simulink library "LopesDevelopmentLibrary"  (R2015b)
settings: Solver=ode45  StartTime=0.0  StopTime=10.0  RelTol=1e-3
values from neighbouring files (symbols this model uses):
  d2r = @(d) d*(pi/180)    [LopesDevelopmentLibrary_LoadParameters.m]
  ts = LopesParams.ts    [LopesDevelopmentLibrary_LoadParameters.m]
undefined symbols (not defined in the file or in its folder): anyParameterChanged, DiscIntNeverNeededParam, gcbh, LAP, LHF, LKF, LopesParams, macaddr, mxpcnetworkconfig, mxpcrtudprx, mxpcrtudptx, patientParametersChanged, port, PX, PZ, RAP, RHF, RKF, SelectorLOPESInSize, StrideTime_s, Time
undefined symbols (not defined in the file): LopesParamsSendDataArrayLen
libraries: LopesDevelopmentLibrary x327, simulink x100, dspmtrx3 x49, xpciplib x6, xpcnetworkbufferlib x5, dspsigops x4, dspstat3 x3, xpcethernetlib x2, visionstatistics x2, xpcseriallib x2, LopesDevelopmentLibraryTest x1, nmc x1
(part 4 of 12)

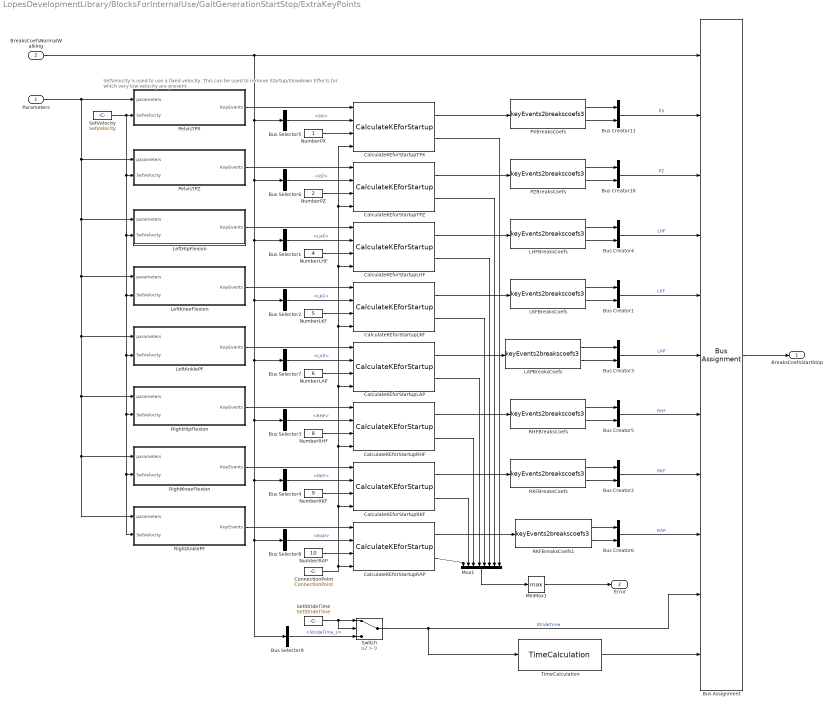
== system LopesDevelopmentLibrary/BlocksForInternalUse/GaitGenerationStartStop/ExtraKeyPoints  ==
  note: SetVelocity is used to use a fixed velocity.
      | This can be used to remove Startup/Slowdown Effects for which very low velocity are present
  Parameters : Inport
  BreaksCoefsNormalWalking : Inport  Port=2
  Bus Creator{1..6,10..11} (8 alike) : BusCreator  Inputs=2
  Bus Selector1 : BusSelector  OutputSignals=LHF
  Bus Selector2 : BusSelector  OutputSignals=LKF
  Bus Selector3 : BusSelector  OutputSignals=RHF
  Bus Selector4 : BusSelector  OutputSignals=RKF
  Bus Selector5 : BusSelector  OutputSignals=PX
  Bus Selector6 : BusSelector  OutputSignals=PZ
  Bus Selector7 : BusSelector  OutputSignals=LAP
  Bus Selector8 : BusSelector  OutputSignals=RAP
  Bus Selector9 : BusSelector  OutputSignals=StrideTime_s
  Bus Assignment : BusAssignment  AssignedSignals=PX,PZ,LHF,LKF,LAP,RHF,RKF,RAP,StrideTime_s,Time
  CalculateKEforStartupLAP : LopesDevelopmentLibrary/BlocksForInternalUse/GaitGenerationStartStop/CalculateKEforStartup
  CalculateKEforStartupLHF : LopesDevelopmentLibrary/BlocksForInternalUse/GaitGenerationStartStop/CalculateKEforStartup
  CalculateKEforStartupLKF : LopesDevelopmentLibrary/BlocksForInternalUse/GaitGenerationStartStop/CalculateKEforStartup
  CalculateKEforStartupRAP : LopesDevelopmentLibrary/BlocksForInternalUse/GaitGenerationStartStop/CalculateKEforStartup
  CalculateKEforStartupRHF : LopesDevelopmentLibrary/BlocksForInternalUse/GaitGenerationStartStop/CalculateKEforStartup
  CalculateKEforStartupRKF : LopesDevelopmentLibrary/BlocksForInternalUse/GaitGenerationStartStop/CalculateKEforStartup
  CalculateKEforStartupTPX : LopesDevelopmentLibrary/BlocksForInternalUse/GaitGenerationStartStop/CalculateKEforStartup
  CalculateKEforStartupTPZ : LopesDevelopmentLibrary/BlocksForInternalUse/GaitGenerationStartStop/CalculateKEforStartup
  ConnectionPoint : Constant  Value=ConnectionPoint
  LAPBreaksCoefs : LopesDevelopmentLibrary/BlocksForInternalUse/GaitGeneration/keyEvents2breakscoefs3  SystemSampleTime=-1
  LHFBreaksCoefs : LopesDevelopmentLibrary/BlocksForInternalUse/GaitGeneration/keyEvents2breakscoefs3  SystemSampleTime=-1
  LKFBreaksCoefs : LopesDevelopmentLibrary/BlocksForInternalUse/GaitGeneration/keyEvents2breakscoefs3  SystemSampleTime=-1
  LeftAnklePF : Subsystem
  LeftHipFlexion : Subsystem
  LeftKneeFlexion : Subsystem
  MinMax1 : MinMax  Function=max
  Mux1 : Mux  Inputs=8
  NumberLAP : Constant  Value=6
  NumberLHF : Constant  Value=4
  NumberLKF : Constant  Value=5
  NumberPX : Constant
  NumberPZ : Constant  Value=2
  NumberRAP : Constant  Value=10
  NumberRHF : Constant  Value=8
  NumberRKF : Constant  Value=9
  PXBreaksCoefs : LopesDevelopmentLibrary/BlocksForInternalUse/GaitGeneration/keyEvents2breakscoefs3  SystemSampleTime=-1
  PZBreaksCoefs : LopesDevelopmentLibrary/BlocksForInternalUse/GaitGeneration/keyEvents2breakscoefs3  SystemSampleTime=-1
  PelvisTPX : Subsystem
  PelvisTPZ : Subsystem
  RHFBreaksCoefs : LopesDevelopmentLibrary/BlocksForInternalUse/GaitGeneration/keyEvents2breakscoefs3  SystemSampleTime=-1
  RKFBreaksCoefs : LopesDevelopmentLibrary/BlocksForInternalUse/GaitGeneration/keyEvents2breakscoefs3  SystemSampleTime=-1
  RKFBreaksCoefs1 : LopesDevelopmentLibrary/BlocksForInternalUse/GaitGeneration/keyEvents2breakscoefs3  SystemSampleTime=-1
  RightAnklePF : Subsystem
  RightHipFlexion : Subsystem
  RightKneeFlexion : Subsystem
  SetStrideTime : Constant  Value=SetStrideTime
  SetVelocity : Constant  Value=SetVelocity
  Switch : Switch  Criteria=u2 > Threshold
  TimeCalculation : LopesDevelopmentLibraryTest/BlocksForInternalUse/GaitGenerationStartStop/ExtraKeyPoints /TimeCalculation
  BreaksCoefsStartStop : Outport
  Error : Outport  Port=2
  wires:
  Switch/1 -> TimeCalculation/1, Bus Assignment/10  "StrideTime"
  BreaksCoefsNormalWalking/1 -> Bus Assignment/1, Bus Selector5/1, Bus Selector6/1, Bus Selector7/1, Bus Selector4/1, Bus Selector8/1, Bus Selector9/1, Bus Selector3/1, Bus Selector2/1, Bus Selector1/1
  Bus Selector9/1 -> Switch/3  "<StrideTime_s>"
  SetStrideTime/1 -> Switch/2, Switch/1
  TimeCalculation/1 -> Bus Assignment/11
  Parameters/1 -> PelvisTPX/1(parameters), PelvisTPZ/1(parameters), LeftHipFlexion/1(parameters), LeftKneeFlexion/1(parameters), LeftAnklePF/1(parameters), RightHipFlexion/1(parameters), RightKneeFlexion/1(parameters), RightAnklePF/1(parameters)
  RightAnklePF/1(KeyEvents) -> CalculateKEforStartupRAP/1
  NumberRAP/1 -> CalculateKEforStartupRAP/3
  Bus Selector8/1 -> CalculateKEforStartupRAP/2  "<RAP>"
  CalculateKEforStartupRAP/1 -> RKFBreaksCoefs1/1
  Bus Creator6/1 -> Bus Assignment/9  "RAP"
  RKFBreaksCoefs1/2 -> Bus Creator6/2
  RKFBreaksCoefs1/1 -> Bus Creator6/1
  Bus Creator3/1 -> Bus Assignment/6  "LAP"
  LAPBreaksCoefs/2 -> Bus Creator3/2
  LAPBreaksCoefs/1 -> Bus Creator3/1
  CalculateKEforStartupLAP/1 -> LAPBreaksCoefs/1
  Bus Selector7/1 -> CalculateKEforStartupLAP/2  "<LAP>"
  LeftAnklePF/1(KeyEvents) -> CalculateKEforStartupLAP/1
  NumberLAP/1 -> CalculateKEforStartupLAP/3
  Bus Assignment/1 -> BreaksCoefsStartStop/1
  ConnectionPoint/1 -> CalculateKEforStartupRKF/4, CalculateKEforStartupLKF/4, CalculateKEforStartupTPX/4, CalculateKEforStartupTPZ/4, CalculateKEforStartupLHF/4, CalculateKEforStartupLAP/4, CalculateKEforStartupRHF/4, CalculateKEforStartupRAP/4
  Bus Creator2/1 -> Bus Assignment/8  "RKF"
  Bus Creator5/1 -> Bus Assignment/7  "RHF"
  Bus Creator1/1 -> Bus Assignment/5  "LKF"
  CalculateKEforStartupLHF/2 -> Mux1/6
  CalculateKEforStartupLKF/2 -> Mux1/5
  CalculateKEforStartupRHF/2 -> Mux1/3
  CalculateKEforStartupRKF/2 -> Mux1/2
  CalculateKEforStartupLHF/1 -> LHFBreaksCoefs/1
  RightKneeFlexion/1(KeyEvents) -> CalculateKEforStartupRKF/1
  LeftKneeFlexion/1(KeyEvents) -> CalculateKEforStartupLKF/1
  RightHipFlexion/1(KeyEvents) -> CalculateKEforStartupRHF/1
  NumberRKF/1 -> CalculateKEforStartupRKF/3
  NumberRHF/1 -> CalculateKEforStartupRHF/3
  NumberLKF/1 -> CalculateKEforStartupLKF/3
  Bus Selector1/1 -> CalculateKEforStartupLHF/2  "<LHF>"
  LeftHipFlexion/1(KeyEvents) -> CalculateKEforStartupLHF/1
  NumberLHF/1 -> CalculateKEforStartupLHF/3
  CalculateKEforStartupRKF/1 -> RKFBreaksCoefs/1
  CalculateKEforStartupLKF/1 -> LKFBreaksCoefs/1
  CalculateKEforStartupRHF/1 -> RHFBreaksCoefs/1
  Bus Creator4/1 -> Bus Assignment/4  "LHF"
  Bus Selector4/1 -> CalculateKEforStartupRKF/2  "<RKF>"
  Bus Selector3/1 -> CalculateKEforStartupRHF/2  "<RHF>"
  Bus Selector2/1 -> CalculateKEforStartupLKF/2  "<LKF>"
  LKFBreaksCoefs/2 -> Bus Creator1/2
  RKFBreaksCoefs/2 -> Bus Creator2/2
  LKFBreaksCoefs/1 -> Bus Creator1/1
  RKFBreaksCoefs/1 -> Bus Creator2/1
  LHFBreaksCoefs/2 -> Bus Creator4/2
  RHFBreaksCoefs/2 -> Bus Creator5/2
  RHFBreaksCoefs/1 -> Bus Creator5/1
  LHFBreaksCoefs/1 -> Bus Creator4/1
  Mux1/1 -> MinMax1/1
  MinMax1/1 -> Error/1
  SetVelocity/1 -> PelvisTPX/2(SetVelocity), PelvisTPZ/2(SetVelocity), LeftAnklePF/2(SetVelocity), RightHipFlexion/2(SetVelocity), RightKneeFlexion/2(SetVelocity), RightAnklePF/2(SetVelocity), LeftKneeFlexion/2(SetVelocity), LeftHipFlexion/2(SetVelocity)
  CalculateKEforStartupTPX/1 -> PXBreaksCoefs/1
  CalculateKEforStartupTPZ/1 -> PZBreaksCoefs/1
  NumberPZ/1 -> CalculateKEforStartupTPZ/3
  PelvisTPX/1(KeyEvents) -> CalculateKEforStartupTPX/1
  PelvisTPZ/1(KeyEvents) -> CalculateKEforStartupTPZ/1
  NumberPX/1 -> CalculateKEforStartupTPX/3
  Bus Selector5/1 -> CalculateKEforStartupTPX/2  "<PX>"
  Bus Selector6/1 -> CalculateKEforStartupTPZ/2  "<PZ>"
  PXBreaksCoefs/1 -> Bus Creator11/1
  PXBreaksCoefs/2 -> Bus Creator11/2
  PZBreaksCoefs/1 -> Bus Creator10/1
  PZBreaksCoefs/2 -> Bus Creator10/2
  Bus Creator10/1 -> Bus Assignment/3  "PZ"
  Bus Creator11/1 -> Bus Assignment/2  "PX"
  CalculateKEforStartupTPZ/2 -> Mux1/7
  CalculateKEforStartupTPX/2 -> Mux1/8
  CalculateKEforStartupRAP/2 -> Mux1/1
  CalculateKEforStartupLAP/2 -> Mux1/4

== system LopesDevelopmentLibrary/BlocksForInternalUse/GaitGenerationStartStop/OrderKeyEventsAddOne ==
  kE : Inport
  JointNumber : Inport  Port=2
  phase : Inport  Port=3
  yy : Inport  Port=4
  dydx : Inport  Port=5
  SortAndAddKeyEvents : MATLAB Function  TreatAsAtomicUnit=on
  kE_out : Outport
  isError : Outport  Port=2
  wires:
  dydx/1 -> SortAndAddKeyEvents/5(dydx)
  yy/1 -> SortAndAddKeyEvents/4(yy)
  phase/1 -> SortAndAddKeyEvents/3(phase)
  SortAndAddKeyEvents/1(kE_out) -> kE_out/1
  SortAndAddKeyEvents/2(Error) -> isError/1
  kE/1 -> SortAndAddKeyEvents/1(kE)
  JointNumber/1 -> SortAndAddKeyEvents/2(jointNumber)

== system LopesDevelopmentLibrary/BlocksForInternalUse/LLC Communication/LLC Network Configuration ==
  note: This block initializes the separate network card in
      | the (real) xPC Target. When built for usage with the
      | Virtual Machine version (LopesUseRealTimeUDP=0),
      | this block does nothing.
  Dummy : Terminator
  Dummy1 : Constant
  Variant Network Init : Subsystem  Variant=on
  wires:
  Variant Network Init/1(Dummy_out) -> Dummy/1
  Dummy1/1 -> Variant Network Init/1(Dummy_in)

== system LopesDevelopmentLibrary/BlocksForInternalUse/LLC Communication/LLCReceiveUDP ==
  Enable : EnablePort
  Constant3 : Constant  Value=uint8(['Recv ',num2str(port),': '])
  Debug : Subsystem
      mask Display: disp('')
  Dummy1 : Constant  Value=0
  EnableDebug : Constant  Value=false  OutDataTypeStr=boolean
      settings: OpenFcn=|
      | b = get_param(gcb,'value');
      | if (strcmp(b,'true')),
      |   set_param (gcb,'value','false');
      | else
      |   set_param(gcb,'value','true');
      | end;
  ShowInMatlabConsoleIfNotEmpty : MATLAB Function  TreatAsAtomicUnit=on
  UDPReceiveVariantChannel : Subsystem  Variant=on
  RecvData : Outport
  RecvLen : Outport  Port=2
  wires:
  Dummy1/1 -> UDPReceiveVariantChannel/1(Dummy_in)
  Constant3/1 -> ShowInMatlabConsoleIfNotEmpty/3(pre)
  UDPReceiveVariantChannel/1(RecvData) -> RecvData/1, ShowInMatlabConsoleIfNotEmpty/1(stringArray)
  EnableDebug/1 -> ShowInMatlabConsoleIfNotEmpty/4(enable)
  UDPReceiveVariantChannel/2(RecvLen) -> RecvLen/1, ShowInMatlabConsoleIfNotEmpty/2(len)

== system LopesDevelopmentLibrary/BlocksForInternalUse/LLC Communication/LLCSendUDP ==
  SendData : Inport
  SendLen : Inport  Port=2
  Enable : EnablePort
  Compare To Zero : simulink/Logic and Bit Operations/Compare To Zero  relop=>  OutDataTypeStr=boolean
  Constant6 : Constant  Value=uint8(['Send ',num2str(port),': '])
  Debug : Subsystem
      mask Display: disp('')
  EnableDebug : Constant  Value=false  OutDataTypeStr=boolean
      settings: OpenFcn=|
      | b = get_param(gcb,'value');
      | if (strcmp(b,'true')),
      |   set_param (gcb,'value','false');
      | else
      |   set_param(gcb,'value','true');
      | end;
  ShowInMatlabConsole IfNotEmpty : MATLAB Function  TreatAsAtomicUnit=on
  UDPSendVariant : Subsystem
  wires:
  Constant6/1 -> ShowInMatlabConsole IfNotEmpty/3(pre)
  EnableDebug/1 -> ShowInMatlabConsole IfNotEmpty/4(enable)
  SendData/1 -> UDPSendVariant/1(Data), ShowInMatlabConsole IfNotEmpty/1(stringArray)
  Compare To Zero/1 -> UDPSendVariant/Enable
  SendLen/1 -> Compare To Zero/1, UDPSendVariant/2(Len), ShowInMatlabConsole IfNotEmpty/2(len)

== system LopesDevelopmentLibrary/BlocksForInternalUse/LLC Communication/UDP_Blocks ==
  note: These blocks are copies of the UDP blocks (as of R2015b: Legacy UDP) for non-realtime and the RealTime UDP blocks of the xPC/SLRT libraries of different Matlab versions. copied them and disabled/broke the links to the original libraries (needed for the second bullet below). They differ from the original blocks in the Library on the following points:
      | I changed the mask. Foar these blocks, the IP address _is_ evaluated (for the standard blocks it is not). This allows for usage of a variable as IP address (it should be a string).I reduced the receive buffering settings so that always the most recent packet is received (the older ones are discarded).
  "Network Configuration_RT_2012b " : Subsystem  mask(xpcnwconfig){IpAddress=LopesParams.Communication.ipSelf_RT, SubnetMask=255.255.255.0, Gateway=0.0.0.0, EthDrv=Intel Gigabit, PciBus=LopesParams.Communication.busSelf_RT, PciSlot=LopesParams.Communication.slotSelf_RT}
      mask prompts: IpAddress "IP Address:"; SubnetMask "Subnet Mask:"; EthDrv "Ethernet Driver"; PciBus "PCI Bus:"; PciSlot "PCI Slot:"
      mask help: Network Configuration
      mask init:
      | IpAddress = ipaddr(IpAddress);
      | SubnetMask = ipaddr(SubnetMask);
      | Gateway = ipaddr(Gateway);
      mask Help: eval('xpcdoc(''RT_NETWORK_CONFIGURATION'')');
      mask TypeOptions EthDrv: Intel 8255x | Intel Gigabit
      mask Display: disp('Network Configuration');
  "Network Configuration_RT_2014b " : Subsystem  InitFcn=mxpcnetworkconfig(1);  mask(xpcnwconfig){ID=1, IpAddress=LopesParams.Communication.ipSelf_RT, SubnetMask=255.255.255.0, Gateway=0.0.0.0, EthDrv=Intel Gigabit, PciBus=LopesParams.Communication.busSelf_RT, PciSlot=LopesParams.Communication.slotSelf_RT, udpID=0}
      mask prompts: ID "Device ID:"; IpAddress "IP Address:"; SubnetMask "Subnet Mask:"; EthDrv "Ethernet Driver:"; PciBus "PCI Bus:"; PciSlot "PCI Slot:"; udpID "Internal UDP ID:"
      mask help: Configure network interface for real-time UDP communication
      mask init:
      | IpAddress = ipaddr(IpAddress);
      | SubnetMask = ipaddr(SubnetMask);
      | Gateway = ipaddr(Gateway);
      | udpID = ID - 1;
      | 
      | [MaskDisplay] = mxpcnetworkconfig(2, ID, EthDrv, PciBus, PciSlot);
      | set_param(gcb, 'MaskDisplay', MaskDisplay);
      mask Help: eval('xpcdoc(''RT_NETWORK_CONFIGURATION'')');
      mask TypeOptions ID: Ethernet Init /ID
      mask TypeOptions EthDrv: Ethernet Init /Driver
      mask Display: disp('Real-time UDP\nConfiguration\nBus: 2 Slot: 4\nId: 1\nIntel Gigabit');
  Network Configuration_RT_2015b : Subsystem  InitFcn=mxpcnetworkconfig(1);  mask(xpcnwconfig){ID=1, IpAddress=LopesParams.Communication.ipSelf_RT, SubnetMask=255.255.255.0, Gateway=0.0.0.0, EthDrv=Intel Gigabit, PciBus=LopesParams.Communication.busSelf_RT, PciSlot=LopesParams.Communication.slotSelf_RT, udpID=0, MulticastList=[], Multicast={}}
      mask prompts: ID "Device ID:"; IpAddress "IP Address:"; SubnetMask "Subnet Mask:"; EthDrv "Ethernet Driver:"; PciBus "PCI Bus:"; PciSlot "PCI Slot:"; udpID "Internal UDP ID:"; MulticastList "[Multicast IP]"; Multicast "Multicast address list:"
      mask help: Configure network interface for real-time UDP communication.
      mask init: same as LopesDevelopmentLibrary/BlocksForInternalUse/LLC Communication/UDP_Blocks/Network Configuration_RT_2014b 
      mask Help: eval('xpcdoc(''RT_NETWORK_CONFIGURATION'')');
      mask TypeOptions ID: Ethernet Init /ID
      mask TypeOptions EthDrv: Ethernet Init /Driver
      mask TypeOptions MulticastList: ARP Init /MulticastList
      mask TypeOptions Multicast: Ethernet Init /Multicast
      mask Display: disp('Real-time UDP\nConfiguration\nBus: 2 Slot: 4\nId: 1\nIntel Gigabit');
  Receive_Non-RT : S-Function  FunctionName=xpcudpbytereceive  Parameters=ipAdd, ipPort, width, sampletime, vblLen  SFunctionDeploymentMode=off  EnableBusSupport=off  mask(xpcudpbytereceive){ipAddress='0.0.0.0', ipPort=port, width=1500, vblLen=on, sampletime=LopesParams.ts}
      mask prompts: ipAddress "IP address to receive from ('0.0.0.0' for accepting all):"; ipPort "IP port to receive from:"; width "Output port width (number of bytes):"; vblLen "Allow variable length packets"; sampletime "Sample time:"
      mask init:
      | %mudp('ipPort', 'IP Port');
      | ipAdd = ipAddressFromString(ipAddress);
      mask Help: eval('xpcdoc(''UDP_Receive'')');
      mask Display: disp('Non-RT\nUDP Recv\nBinary')
  "Receive_RT_2012b " : Subsystem  mask(receive){Receive1='0.0.0.0', Receive2=port, Receive3=1500, Receive4=LopesParams.ts}
      mask prompts: Receive1 "IP address to receive from ('0.0.0.0' for accepting all):"; Receive2 "IP port to receive from:"; Receive3 "Output port width:"; Receive4 "Sample time:"
      mask init:
      | Receive1 = ipaddr(Receive1);
      mask Help: helpview(fullfile(docroot, 'mapfiles', 'xpc.map'), 'RT_UDP_RECEIVE')
      mask Display: disp('RT UDP\nReceive')
  "Receive_RT_2014b " : Subsystem  InitFcn=mxpcrtudprx(1, get_param(gcbh, 'ID'));  mask(rtudpreceive){ID=1, Receive1='0.0.0.0', Receive2=port, Receive3=1500, Receive4=LopesParams.ts, udpID=0}
      mask prompts: ID "Device ID:"; Receive1 "Source IP Address:"; Receive2 "Local (destination) port:"; Receive3 "Output port width:"; Receive4 "Sample time:"; udpID "Internal UDP ID:"
      mask help:
      | Receive data over UDP network.
      |
      | This block receives data on the specified local (destination) port. To receive all data sent to this port, set 'Source IP Address' to 0.0.0.0. To receive data sent to this port from a specific remote source, enter that IP address.
      mask init:
      | Receive1 = ipaddr(Receive1);
      | udpID = ID -1;
      | [MaskDisplay] = mxpcrtudprx(2, ID);
      | set_param(gcb, 'MaskDisplay', MaskDisplay);
      mask Help: eval('xpcdoc(''RT_UDP_RECEIVE'')');
      mask TypeOptions ID: 1 | 2 | 3 | 4 | 5 | 6 | 7 | 8
      mask Display:
      | disp('UDP\nReceive\nId: 1');
      | port_label('output', 1, 'Data');
      | port_label('output', 2, 'N');
  Receive_RT_2015b : Subsystem  InitFcn=mxpcrtudprx(1, get_param(gcbh, 'ID'));  mask(rtudpreceive){ID=1, Receive1='0.0.0.0', Receive2=port, Receive3=1500, Receive4=LopesParams.ts, udpID=0}
      mask prompts: ID "Device ID:"; Receive1 "Source IP Address:"; Receive2 "Local (destination) port:"; Receive3 "Output port width:"; Receive4 "Sample time:"; udpID "Internal UDP ID:"
      mask help:
      | Receive data over UDP network on a dedicated network interface.
      |
      | This block receives data on the specified local (destination) port. To receive all data sent to this port, set 'Source IP Address' to 0.0.0.0. To receive data sent to this port from a specific remote source, enter the IP address of that source.
      mask init:
      | Receive1 = ipaddr(Receive1);
      | udpID = ID -1;
      | [MaskDisplay] = mxpcrtudprx(2, ID);
      | set_param(gcb, 'MaskDisplay', MaskDisplay);
      mask Help: eval('xpcdoc(''RT_UDP_RECEIVE'')');
      mask TypeOptions ID: 1 | 2 | 3 | 4 | 5 | 6 | 7 | 8
      mask Display:
      | disp('UDP\nReceive\nId: 1');
      | port_label('output', 1, 'Data');
      | port_label('output', 2, 'N');
  Send_Non-RT : S-Function  FunctionName=xpcudpbytesend  Parameters=ipAdd, ipPort, localPort, sampletime, vblLen  SFunctionDeploymentMode=off  EnableBusSupport=off  mask(xpcudpbytesend){ipAddress=LopesParams.Communication.ipLLC_NonRT, ipPort=port, localPort=-1, vblLen=on, sampletime=LopesParams.ts}
      mask prompts: ipAddress "IP address to send to ('255.255.255.255' for broadcast):"; ipPort "Remote IP port to send to:"; localPort "Use the following local IP port (-1 for automatic port assignment):"; vblLen "Allow variable length packets"; sampletime "Sample time:"
      mask init:
      | if localPort ~= -1
      |   mudp('localPort', 'Local IP Port');
      | end
      | ipAdd = ipAddressFromString(ipAddress);
      mask Help: eval('xpcdoc(''UDP_Send'')');
      mask Display: disp('Non-RT\nUDP Send\nBinary')
  Send_RT_2012b : Subsystem  mask(send){Send1=LopesParams.Communication.ipLLC_RT, Send2=port, Send3=-1, Send4=LopesParams.ts}
      mask prompts: Send1 "IP address to send to ('255.255.255.255' for broadcast):"; Send2 "Remote IP port to send to:"; Send3 "Use the following local IP port (-1 for automatic assignment):"; Send4 "Sample time:"
      mask init:
      | Send1 = ipaddr(Send1);
      mask Help: helpview(fullfile(docroot, 'mapfiles', 'xpc.map'), 'RT_UDP_SEND')
      mask Display: disp('RT UDP\nSend')
  Send_RT_2014b : Subsystem  InitFcn=mxpcrtudptx(1, get_param(gcbh, 'ID'));  mask(rtudpsend){ID=1, Send1=LopesParams.Communication.ipLLC_RT, Send2=port, Send3=-1, Send4=LopesParams.ts, udpID=0}
      mask prompts: ID "Device ID:"; Send1 "Destination IP address:"; Send2 "Destination port:"; Send3 "Local (source) port:"; Send4 "Sample time:"; udpID "Internal UDP ID:"
      mask help:
      | Send data over UDP network.
      |
      | This block sends data from the 'Local (source) port' to the 'Destination port'. To broadcast data to 'Destination port' on all devices set 'Destination IP Address' to 255.255.255.255. To send data to a specific remote destintion set that IP address. Set 'Local (source) port' to -1 for automatic assignment.
      mask init:
      | Send1 = ipaddr(Send1);
      | udpID = ID -1;
      | MaskDisplay = mxpcrtudptx(2, ID);
      | set_param(gcb, 'MaskDisplay', MaskDisplay);
      mask Help: eval('xpcdoc(''RT_UDP_SEND'')');
      mask TypeOptions ID: 1 | 2 | 3 | 4 | 5 | 6 | 7 | 8
      mask Display:
      | disp('UDP\nSend\nId: 1');
      | port_label('input', 1, 'Data');
      | port_label('input', 2, 'N');
  Send_RT_2015b : Subsystem  InitFcn=mxpcrtudptx(1, get_param(gcbh, 'ID'));  mask(rtudpsend){ID=1, Send1=LopesParams.Communication.ipLLC_RT, Send2=port, Send3=-1, Send4=LopesParams.ts, udpID=0}
      mask prompts: ID "Device ID:"; Send1 "Destination IP address:"; Send2 "Destination port:"; Send3 "Local (source) port:"; Send4 "Sample time:"; udpID "Internal UDP ID:"
      mask help:
      | Send data over UDP network on a dedicated network interface.
      |
      | This block sends data from the 'Local (source) port' to the 'Destination port'. To broadcast data to 'Destination port' on all devices set 'Destination IP Address' to 255.255.255.255. To send data to a specific remote destintion set that IP address. Set 'Local (source) port' to -1 for automatic assignment.
      mask init:
      | Send1 = ipaddr(Send1);
      | udpID = ID -1;
      | MaskDisplay = mxpcrtudptx(2, ID);
      | set_param(gcb, 'MaskDisplay', MaskDisplay);
      mask Help: eval('xpcdoc(''RT_UDP_SEND'')');
      mask TypeOptions ID: 1 | 2 | 3 | 4 | 5 | 6 | 7 | 8
      mask Display:
      | disp('UDP\nSend\nId: 1');
      | port_label('input', 1, 'Data');
      | port_label('input', 2, 'N');

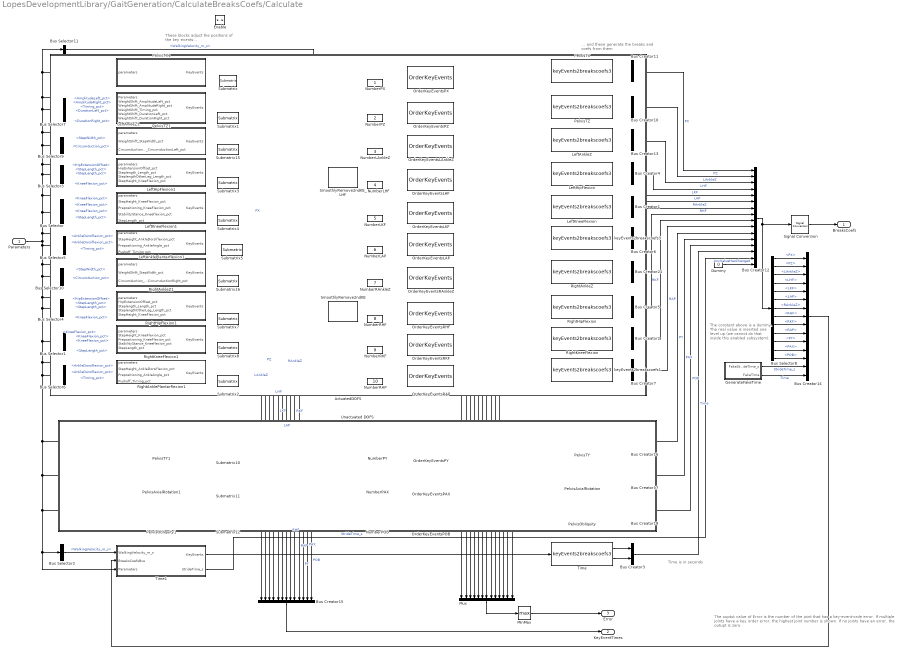
== system LopesDevelopmentLibrary/GaitGeneration/CalculateBreaksCoefs/Calculate ==
  note: The ouptut value of Error is the number of the joint that has a key-event-orde  error.
      | If multiple joints have a key order error, the highest joint number is shown. If
      | no joints have an error, the outupt is zero.
  note: The constant above is
      | a dummy. The real value
      | is inserted one level up
      | (we cannot do that inside this
      | enabled subsystem).
  note: These blocks adjust the positions
      | of the key events...
  note: ... and these generate the breaks
      | and coefs from them
  note: Time is in seconds
  Parameters : Inport
  Enable : EnablePort
  ActuatedDOFS : Subsystem
      mask Display: disp('')
  Bus Creator{1..7,10..11,13,16..18,21} (14 alike) : BusCreator  Inputs=2
  Bus Creator12 : BusCreator  Inputs=16
  Bus Creator14 : BusCreator  Inputs=15
  Bus Creator15 : BusCreator  Inputs=13
  Bus Selector : BusSelector  OutputSignals=LeftStepHeight.KneeFlexion_pct,LeftPrepositioning.KneeFlexion_pct,LeftStabilityStance.KneeFlexion_pct,LeftSteplength.StepLength_pct
  Bus Selector1 : BusSelector  OutputSignals=RightStepHeight.KneeFlexion_pct,RightPrepositioning.KneeFlexion_pct,RightStabilityStance.KneeFlexion_pct,RightSteplength.StepLength_pct
  Bus Selector10 : BusSelector  OutputSignals=WeightShift.StepWidth_pct,RightCircumduction.Circumduction_pct
  Bus Selector11 : BusSelector  OutputSignals=General.WalkingVelocity_m_s
  Bus Selector2 : BusSelector  OutputSignals=General.WalkingVelocity_m_s
  Bus Selector3 : BusSelector  OutputSignals=General.HipExtensionOffset,LeftSteplength.StepLength_pct,RightSteplength.StepLength_pct,LeftStepHeight.KneeFlexion_pct
  Bus Selector4 : BusSelector  OutputSignals=General.HipExtensionOffset,RightSteplength.StepLength_pct,LeftSteplength.StepLength_pct,RightStepHeight.KneeFlexion_pct
  Bus Selector5 : BusSelector  OutputSignals=LeftStepHeight.AnkleDorsiflexion_pct,LeftPrepositioning.AnkleDorsiflexion_pct,LeftPushoff.Timing_pct
  Bus Selector6 : BusSelector  OutputSignals=RightStepHeight.AnkleDorsiflexion_pct,RightPrepositioning.AnkleDorsiflexion_pct,RightPushoff.Timing_pct
  Bus Selector7 : BusSelector  OutputSignals=WeightShift.AmplitudeLeft_pct,WeightShift.AmplitudeRight_pct,WeightShift.Timing_pct,WeightShift.DurationLeft_pct,WeightShift.DurationRight_pct
  Bus Selector8 : BusSelector  OutputSignals=PX,PZ,LAnkleZ,LHF,LKF,LAP,RAnkleZ,RHF,RKF,RAP,PY,PAX,POB
  Bus Selector9 : BusSelector  OutputSignals=WeightShift.StepWidth_pct,LeftCircumduction.Circumduction_pct
  Dummy : Constant  Value=0  OutDataTypeStr=double
  GenerateFakeTime : Subsystem
  LeftAnklePlantarflexion1 : Subsystem
  LeftAnkleZ : LopesDevelopmentLibrary/BlocksForInternalUse/GaitGeneration/keyEvents2breakscoefs3  SystemSampleTime=-1
  LeftAnkleZ1 : Subsystem
  LeftHipFlexion : LopesDevelopmentLibrary/BlocksForInternalUse/GaitGeneration/keyEvents2breakscoefs3  SystemSampleTime=-1
  LeftHipFlexion1 : Subsystem
  LeftKneeFlexion : LopesDevelopmentLibrary/BlocksForInternalUse/GaitGeneration/keyEvents2breakscoefs3  SystemSampleTime=-1
  LeftKneeFlexion1 : Subsystem
  MinMax : MinMax  Function=max
  Mux : Mux  Inputs=13
  NumberLAP : Constant  Value=6
  NumberLAnkleZ : Constant  Value=3
  NumberLHF : Constant  Value=4
  NumberLKF : Constant  Value=5
  NumberPAX : Constant  Value=12
  NumberPOB : Constant  Value=13
  NumberPX : Constant
  NumberPY : Constant  Value=11
  NumberPZ : Constant  Value=2
  NumberRAP : Constant  Value=10
  NumberRAnkleZ : Constant  Value=7
  NumberRHF : Constant  Value=8
  NumberRKF : Constant  Value=9
  OrderKeyEventsLAP : LopesDevelopmentLibrary/BlocksForInternalUse/GaitGeneration/OrderKeyEvents
  OrderKeyEventsLAnkleZ : LopesDevelopmentLibrary/BlocksForInternalUse/GaitGeneration/OrderKeyEvents
  OrderKeyEventsLHF : LopesDevelopmentLibrary/BlocksForInternalUse/GaitGeneration/OrderKeyEvents
  OrderKeyEventsLKF : LopesDevelopmentLibrary/BlocksForInternalUse/GaitGeneration/OrderKeyEvents
  OrderKeyEventsPAX : LopesDevelopmentLibrary/BlocksForInternalUse/GaitGeneration/OrderKeyEvents
  OrderKeyEventsPOB : LopesDevelopmentLibrary/BlocksForInternalUse/GaitGeneration/OrderKeyEvents
  OrderKeyEventsPX : LopesDevelopmentLibrary/BlocksForInternalUse/GaitGeneration/OrderKeyEvents
  OrderKeyEventsPY : LopesDevelopmentLibrary/BlocksForInternalUse/GaitGeneration/OrderKeyEvents
  OrderKeyEventsPZ : LopesDevelopmentLibrary/BlocksForInternalUse/GaitGeneration/OrderKeyEvents
  OrderKeyEventsRAP : LopesDevelopmentLibrary/BlocksForInternalUse/GaitGeneration/OrderKeyEvents
  OrderKeyEventsRAnkleZ : LopesDevelopmentLibrary/BlocksForInternalUse/GaitGeneration/OrderKeyEvents
  OrderKeyEventsRHF : LopesDevelopmentLibrary/BlocksForInternalUse/GaitGeneration/OrderKeyEvents
  OrderKeyEventsRKF : LopesDevelopmentLibrary/BlocksForInternalUse/GaitGeneration/OrderKeyEvents
  PelvisAxialRotation : LopesDevelopmentLibrary/BlocksForInternalUse/GaitGeneration/keyEvents2breakscoefs3  SystemSampleTime=-1
  PelvisAxialRotation1 : Subsystem
  PelvisObliquity : LopesDevelopmentLibrary/BlocksForInternalUse/GaitGeneration/keyEvents2breakscoefs3  SystemSampleTime=-1
  PelvisObliquity1 : Subsystem
  PelvisTX : LopesDevelopmentLibrary/BlocksForInternalUse/GaitGeneration/keyEvents2breakscoefs3  SystemSampleTime=-1
  PelvisTX1 : Subsystem
  PelvisTY : LopesDevelopmentLibrary/BlocksForInternalUse/GaitGeneration/keyEvents2breakscoefs3  SystemSampleTime=-1
  PelvisTY1 : Subsystem
  PelvisTZ : LopesDevelopmentLibrary/BlocksForInternalUse/GaitGeneration/keyEvents2breakscoefs3  SystemSampleTime=-1
  PelvisTZ1 : Subsystem
  RightAnklePlantarflexion1 : Subsystem
  RightAnkleZ : LopesDevelopmentLibrary/BlocksForInternalUse/GaitGeneration/keyEvents2breakscoefs3  SystemSampleTime=-1
  RightAnkleZ1 : Subsystem
  RightHipFlexion : LopesDevelopmentLibrary/BlocksForInternalUse/GaitGeneration/keyEvents2breakscoefs3  SystemSampleTime=-1
  RightHipFlexion1 : Subsystem
  RightKneeFlexion : LopesDevelopmentLibrary/BlocksForInternalUse/GaitGeneration/keyEvents2breakscoefs3  SystemSampleTime=-1
  RightKneeFlexion1 : Subsystem
  Signal Conversion : SignalConversion
  SmoothlyRemove2ndKE : LopesDevelopmentLibrary/BlocksForInternalUse/GaitGeneration/SmoothlyRemove2ndKE
  SmoothlyRemove2ndKE_LHF : LopesDevelopmentLibrary/BlocksForInternalUse/GaitGeneration/SmoothlyRemove2ndKE
  Submatrix{,1..5,7..8,10..12,15..16} (13 alike) : dspmtrx3/Submatrix  RowSpan=All rows  RowStartMode=First  RowStartIndex=1  RowEndMode=Last  RowEndIndex=1  ColSpan=One column  ColStartMode=First  ColStartIndex=1  ColEndMode=Last  ColEndIndex=1
  Time : LopesDevelopmentLibrary/BlocksForInternalUse/GaitGeneration/keyEvents2breakscoefs3  SystemSampleTime=-1
  Time1 : Subsystem
  Unactuated DOFS : Subsystem
      mask Display: disp('')
  keyEvents2breakscoefs1 : LopesDevelopmentLibrary/BlocksForInternalUse/GaitGeneration/keyEvents2breakscoefs3  SystemSampleTime=-1
  keyEvents2breakscoefs3 : LopesDevelopmentLibrary/BlocksForInternalUse/GaitGeneration/keyEvents2breakscoefs3  SystemSampleTime=-1
  BreaksCoefs : Outport  InitialOutput=0
  KeyEventTimes : Outport  Port=2
  Error : Outport  Port=3
  wires:
  Signal Conversion/1 -> BreaksCoefs/1
  OrderKeyEventsRKF/1 -> RightKneeFlexion/1
  OrderKeyEventsLHF/1 -> LeftHipFlexion/1
  Bus Selector7/5 -> PelvisTZ1/6(WeightShift_DurationRight_pct)  "<DurationRight_pct>"
  LeftHipFlexion1/1(KeyEvents) -> SmoothlyRemove2ndKE_LHF/1, Submatrix3/1
  LeftKneeFlexion/2 -> Bus Creator1/2
  LeftHipFlexion/1 -> Bus Creator4/1
  NumberRHF/1 -> OrderKeyEventsRHF/2
  LeftKneeFlexion/1 -> Bus Creator1/1
  MinMax/1 -> Error/1
  NumberRAnkleZ/1 -> OrderKeyEventsRAnkleZ/2
  OrderKeyEventsPOB/1 -> PelvisObliquity/1
  NumberLHF/1 -> OrderKeyEventsLHF/2
  OrderKeyEventsPY/1 -> PelvisTY/1
  NumberPZ/1 -> OrderKeyEventsPZ/2
  OrderKeyEventsPAX/1 -> PelvisAxialRotation/1
  LeftHipFlexion/2 -> Bus Creator4/2
  NumberLKF/1 -> OrderKeyEventsLKF/2
  Bus Selector3/4 -> LeftHipFlexion1/5(StepHeight_KneeFlexion_pct)  "<KneeFlexion_pct>"
  NumberRKF/1 -> OrderKeyEventsRKF/2
  Bus Selector3/3 -> LeftHipFlexion1/4(SteplengthOtherLeg_Length_pct)  "<StepLength_pct>"
  Bus Selector3/2 -> LeftHipFlexion1/3(Steplength_Length_pct)  "<StepLength_pct>"
  Dummy/1 -> Bus Creator12/16  "AnyValueHasChanged"
  RightHipFlexion1/1(KeyEvents) -> Submatrix7/1, SmoothlyRemove2ndKE/1
  Parameters/1 -> Bus Selector5/1, RightAnklePlantarflexion1/1(parameters), Bus Selector6/1, Time1/3(Parameters), Bus Selector2/1, PelvisObliquity1/1(parameters), PelvisAxialRotation1/1(parameters), PelvisTY1/1(parameters), Bus Selector1/1, Bus Selector4/1, RightHipFlexion1/1(parameters), RightKneeFlexion1/1(parameters), Bus Selector10/1, RightAnkleZ1/1(parameters), LeftAnklePlantarflexion1/1(parameters), Bus Selector11/1, PelvisTX1/1(parameters), PelvisTZ1/1(Parameters), Bus Selector7/1, LeftAnkleZ1/1(parameters), Bus Selector9/1, LeftHipFlexion1/1(parameters), Bus Selector3/1, LeftKneeFlexion1/1(parameters), Bus Selector/1
  RightKneeFlexion1/1(KeyEvents) -> OrderKeyEventsRKF/1, Submatrix8/1
  PelvisTX/2 -> Bus Creator11/2
  Bus Creator12/1 -> Signal Conversion/1, Bus Selector8/1
  Bus Creator2/1 -> Bus Creator12/9  "RKF"
  PelvisTX/1 -> Bus Creator11/1
  Bus Creator1/1 -> Bus Creator12/5  "LKF"
  RightHipFlexion/2 -> Bus Creator5/2
  GenerateFakeTime/1(FakeStrideTime_s) -> Bus Creator14/14  "StrideTime_s"
  Bus Selector7/3 -> PelvisTZ1/4(WeightShift_Timing_pct)  "<Timing_pct>"
  LeftKneeFlexion1/1(KeyEvents) -> OrderKeyEventsLKF/1, Submatrix4/1
  Bus Selector7/1 -> PelvisTZ1/2(WeightShift_AmplitudeLeft_pct)  "<AmplitudeLeft_pct>"
  Bus Creator5/1 -> Bus Creator12/8  "RHF"
  Bus Selector7/4 -> PelvisTZ1/5(WeightShift_DurationLeft_pct)  "<DurationLeft_pct>"
  Bus Selector/1 -> LeftKneeFlexion1/2(StepHeight_KneeFlexion_pct)  "<KneeFlexion_pct>"
  Bus Selector4/4 -> RightHipFlexion1/5(StepHeight_KneeFlexion_pct)  "<KneeFlexion_pct>"
  PelvisTX1/1(KeyEvents) -> Submatrix/1, OrderKeyEventsPX/1
  Bus Creator15/1 -> KeyEventTimes/1
  Bus Creator10/1 -> Bus Creator12/2  "PZ"
  Bus Creator11/1 -> Bus Creator12/1  "PX"
  Bus Creator4/1 -> Bus Creator12/4  "LHF"
  Bus Selector4/3 -> RightHipFlexion1/4(SteplengthOtherLeg_Length_pct)  "<StepLength_pct>"
  Bus Selector4/2 -> RightHipFlexion1/3(Steplength_Length_pct)  "<StepLength_pct>"
  PelvisTZ1/1(KeyEvents) -> OrderKeyEventsPZ/1, Submatrix1/1
  PelvisTZ/1 -> Bus Creator10/1
  PelvisTZ/2 -> Bus Creator10/2
  Bus Selector1/4 -> RightKneeFlexion1/5(StepLength_pct)  "<StepLength_pct>"
  SmoothlyRemove2ndKE/1 -> OrderKeyEventsRHF/1
  Bus Selector4/1 -> RightHipFlexion1/2(HipExtensionOffset_pct)  "<HipExtensionOffset>"
  Submatrix10/1 -> Bus Creator15/11  "PY"
  Time1/2(StrideTime_s) -> Bus Creator12/15  "StrideTime_s"
  SmoothlyRemove2ndKE_LHF/1 -> OrderKeyEventsLHF/1
  Bus Selector3/1 -> LeftHipFlexion1/2(HipExtensionOffset_pct)  "<HipExtensionOffset>"
  Bus Selector1/3 -> RightKneeFlexion1/4(StabilityStance_Kneeflexion_pct)  "<KneeFlexion_pct>"
  Bus Selector1/1 -> RightKneeFlexion1/2(StepHeight_KneeFlexion_pct)  "<KneeFlexion_pct>"
  Bus Selector9/2 -> LeftAnkleZ1/3(Circumduction_CircumductionLeft_pct)  "<Circumduction_pct>"
  Bus Selector9/1 -> LeftAnkleZ1/2(WeightShift_StepWidth_pct)  "<StepWidth_pct>"
  NumberLAnkleZ/1 -> OrderKeyEventsLAnkleZ/2
  Bus Selector8/1 -> Bus Creator14/1  "<PX>"
  Bus Selector10/1 -> RightAnkleZ1/2(WeightShift_StepWidth_pct)  "<StepWidth_pct>"
  NumberPX/1 -> OrderKeyEventsPX/2
  Bus Selector10/2 -> RightAnkleZ1/3(Circumduction_CircumductionRight_pct)  "<Circumduction_pct>"
  Bus Selector/4 -> LeftKneeFlexion1/5(StepLength_pct)  "<StepLength_pct>"
  OrderKeyEventsRAnkleZ/1 -> RightAnkleZ/1
  Bus Creator21/1 -> Bus Creator12/7  "RAnkleZ"
  Bus Selector1/2 -> RightKneeFlexion1/3(Prepositioning_KneeFlexion_pct)  "<KneeFlexion_pct>"
  Mux/1 -> MinMax/1
  Bus Selector7/2 -> PelvisTZ1/3(WeightShift_AmplitudeRight_pct)  "<AmplitudeRight_pct>"
  Bus Selector/2 -> LeftKneeFlexion1/3(Prepositioning_KneeFlexion_pct)  "<KneeFlexion_pct>"
  Bus Creator13/1 -> Bus Creator12/3  "LAnkleZ"
  Bus Selector8/2 -> Bus Creator14/2  "<PZ>"
  Bus Selector/3 -> LeftKneeFlexion1/4(StabilityStance_Kneeflexion_pct)  "<KneeFlexion_pct>"
  Bus Selector8/8 -> Bus Creator14/8  "<RHF>"
  LeftAnkleZ/2 -> Bus Creator13/2
  LeftAnkleZ1/1(KeyEvents) -> Submatrix15/1, OrderKeyEventsLAnkleZ/1
  LeftAnkleZ/1 -> Bus Creator13/1
  RightAnkleZ/2 -> Bus Creator21/2
  RightAnkleZ/1 -> Bus Creator21/1
  RightAnkleZ1/1(KeyEvents) -> Submatrix16/1, OrderKeyEventsRAnkleZ/1
  Bus Selector8/12 -> Bus Creator14/12  "<PAX>"
  OrderKeyEventsLAnkleZ/1 -> LeftAnkleZ/1
  Submatrix11/1 -> Bus Creator15/12  "PAX"
  Time/1 -> Bus Creator3/1
  PelvisTY/1 -> Bus Creator16/1
  Bus Selector8/4 -> Bus Creator14/4  "<LHF>"
  Bus Selector8/7 -> Bus Creator14/7  "<RAnkleZ>"
  Bus Selector8/11 -> Bus Creator14/11  "<PY>"
  OrderKeyEventsLAnkleZ/2 -> Mux/3
  Bus Selector8/13 -> Bus Creator14/13  "<POB>"
  Submatrix12/1 -> Bus Creator15/13  "POB"
  Bus Selector8/9 -> Bus Creator14/9  "<RKF>"
  Submatrix8/1 -> Bus Creator15/9  "RKF"
  Submatrix7/1 -> Bus Creator15/8  "RHF"
  Bus Selector8/5 -> Bus Creator14/5  "<LKF>"
  PelvisObliquity1/1(KeyEvents) -> Submatrix12/1, OrderKeyEventsPOB/1
  Bus Selector11/1 -> SmoothlyRemove2ndKE/2, SmoothlyRemove2ndKE_LHF/2  "<WalkingVelocity_m_s>"
  PelvisTY1/1(KeyEvents) -> OrderKeyEventsPY/1, Submatrix10/1
  OrderKeyEventsPZ/2 -> Mux/2
  Submatrix16/1 -> Bus Creator15/7  "RAnkleZ"
  GenerateFakeTime/2(FakeTime) -> Bus Creator14/15  "Time"
  OrderKeyEventsRHF/2 -> Mux/8
  NumberPOB/1 -> OrderKeyEventsPOB/2
  OrderKeyEventsLKF/2 -> Mux/5
  NumberPY/1 -> OrderKeyEventsPY/2
  OrderKeyEventsRAnkleZ/2 -> Mux/7
  Bus Creator16/1 -> Bus Creator12/11  "PY"
  Submatrix/1 -> Bus Creator15/1  "PX"
  Submatrix15/1 -> Bus Creator15/3  "LAnkleZ"
  Submatrix3/1 -> Bus Creator15/4  "LHF"
  Submatrix1/1 -> Bus Creator15/2  "PZ"
  OrderKeyEventsLHF/2 -> Mux/4
  Submatrix4/1 -> Bus Creator15/5  "LKF"
  OrderKeyEventsRKF/2 -> Mux/9
  OrderKeyEventsPY/2 -> Mux/11
  OrderKeyEventsPOB/2 -> Mux/13
  OrderKeyEventsPX/2 -> Mux/1
  OrderKeyEventsPAX/2 -> Mux/12
  Bus Selector8/3 -> Bus Creator14/3  "<LAnkleZ>"
  PelvisTY/2 -> Bus Creator16/2
  OrderKeyEventsRHF/1 -> RightHipFlexion/1
  Time/2 -> Bus Creator3/2
  Bus Creator14/1 -> Time1/2(BreaksCoefsBus)
  RightHipFlexion/1 -> Bus Creator5/1
  OrderKeyEventsPX/1 -> PelvisTX/1
  OrderKeyEventsLKF/1 -> LeftKneeFlexion/1
  OrderKeyEventsPZ/1 -> PelvisTZ/1
  RightKneeFlexion/1 -> Bus Creator2/1
  Time1/1(KeyEvents) -> Time/1
  Bus Selector2/1 -> Time1/1(WalkingVelocity_m_s)  "<WalkingVelocity_m_s>"
  RightKneeFlexion/2 -> Bus Creator2/2
  PelvisObliquity/2 -> Bus Creator18/2
  Bus Creator17/1 -> Bus Creator12/12  "PAX"
  PelvisAxialRotation1/1(KeyEvents) -> Submatrix11/1, OrderKeyEventsPAX/1
  PelvisAxialRotation/2 -> Bus Creator17/2
  PelvisAxialRotation/1 -> Bus Creator17/1
  NumberPAX/1 -> OrderKeyEventsPAX/2
  Bus Creator18/1 -> Bus Creator12/13  "POB"
  PelvisObliquity/1 -> Bus Creator18/1
  Bus Creator3/1 -> Bus Creator12/14  "Time"
  OrderKeyEventsLAP/1 -> keyEvents2breakscoefs3/1
  OrderKeyEventsRAP/1 -> keyEvents2breakscoefs1/1
  keyEvents2breakscoefs3/1 -> Bus Creator6/1
  keyEvents2breakscoefs3/2 -> Bus Creator6/2
  Bus Creator6/1 -> Bus Creator12/6  "LAP"
  keyEvents2breakscoefs1/2 -> Bus Creator7/2
  keyEvents2breakscoefs1/1 -> Bus Creator7/1
  Bus Creator7/1 -> Bus Creator12/10  "RAP"
  Bus Selector8/10 -> Bus Creator14/10  "<RAP>"
  Bus Selector8/6 -> Bus Creator14/6  "<LAP>"
  OrderKeyEventsRAP/2 -> Mux/10
  OrderKeyEventsLAP/2 -> Mux/6
  NumberLAP/1 -> OrderKeyEventsLAP/2
  NumberRAP/1 -> OrderKeyEventsRAP/2
  RightAnklePlantarflexion1/1(KeyEvents) -> Submatrix2/1, OrderKeyEventsRAP/1
  Submatrix2/1 -> Bus Creator15/10  "RAP"
  LeftAnklePlantarflexion1/1(KeyEvents) -> OrderKeyEventsLAP/1, Submatrix5/1
  Submatrix5/1 -> Bus Creator15/6  "LAP"
  Bus Selector5/1 -> LeftAnklePlantarflexion1/2(StepHeight_AnkleDorsiflexion_pct)  "<AnkleDorsiflexion_pct>"
  Bus Selector5/2 -> LeftAnklePlantarflexion1/3(Prepositioning_AnkleAngle_pct)  "<AnkleDorsiflexion_pct>"
  Bus Selector5/3 -> LeftAnklePlantarflexion1/4(Pushoff_Timing_pct)  "<Timing_pct>"
  Bus Selector6/3 -> RightAnklePlantarflexion1/4(Pushoff_Timing_pct)  "<Timing_pct>"
  Bus Selector6/2 -> RightAnklePlantarflexion1/3(Prepositioning_AnkleAngle_pct)  "<AnkleDorsiflexion_pct>"
  Bus Selector6/1 -> RightAnklePlantarflexion1/2(StepHeight_AnkleDorsiflexion_pct)  "<AnkleDorsiflexion_pct>"

== system LopesDevelopmentLibrary/GaitGeneration/CalculateReferenceStiffnesses/LAP ==
  General_GuidanceForce : Inport
  breaks : Inport  Port=2
  phase : Inport  Port=3
  StepHeight_GuidanceForce : Inport  Port=4
  FootPlacement_GuidanceForce : Inport  Port=5
  PushOff_GuidanceForce : Inport  Port=6
  CalculateStiffnessForOneJoint : LopesDevelopmentLibrary/BlocksForInternalUse/GaitGeneration/CalculateStiffnessForOneJoint
  Constant : Constant  Value=LopesParams.GaitData.StiffnessParameters.AP_StepHeight
  Constant1 : Constant  Value=LopesParams.GaitData.StiffnessParameters.AP_FootPlacement
  Constant2 : Constant  Value=LopesParams.GaitData.StiffnessParameters.AP_PushOff
  Mux : Mux  Inputs=3
  Mux1 : Mux  Inputs=3
  TrajectoryOfInfluence : LopesDevelopmentLibrary/BlocksForInternalUse/GaitGeneration/TrajectoryOfInfluence
  TrajectoryOfInfluence1 : LopesDevelopmentLibrary/BlocksForInternalUse/GaitGeneration/TrajectoryOfInfluence
  TrajectoryOfInfluence2 : LopesDevelopmentLibrary/BlocksForInternalUse/GaitGeneration/TrajectoryOfInfluence
  Stiffness_pct : Outport
  wires:
  Mux/1 -> CalculateStiffnessForOneJoint/2
  PushOff_GuidanceForce/1 -> Mux1/3
  Constant2/1 -> TrajectoryOfInfluence2/1
  TrajectoryOfInfluence2/1 -> Mux/3
  FootPlacement_GuidanceForce/1 -> Mux1/2
  Constant1/1 -> TrajectoryOfInfluence1/1
  Mux1/1 -> CalculateStiffnessForOneJoint/3
  TrajectoryOfInfluence1/1 -> Mux/2
  TrajectoryOfInfluence/1 -> Mux/1
  General_GuidanceForce/1 -> CalculateStiffnessForOneJoint/1
  CalculateStiffnessForOneJoint/1 -> Stiffness_pct/1
  StepHeight_GuidanceForce/1 -> Mux1/1
  Constant/1 -> TrajectoryOfInfluence/1
  breaks/1 -> TrajectoryOfInfluence/2, TrajectoryOfInfluence2/2, TrajectoryOfInfluence1/2
  phase/1 -> TrajectoryOfInfluence/3, TrajectoryOfInfluence2/3, TrajectoryOfInfluence1/3

== system LopesDevelopmentLibrary/GaitGeneration/CalculateReferenceStiffnesses/LHA ==
  WeightShift_GuidanceForce : Inport
  Stiffness_pct : Outport
  wires:
  WeightShift_GuidanceForce/1 -> Stiffness_pct/1

== system LopesDevelopmentLibrary/GaitGeneration/CalculateReferenceStiffnesses/LHA1 ==
  General_GuidanceForce : Inport
  breaks : Inport  Port=2
  phase : Inport  Port=3
  WeightShift_GuidanceForce : Inport  Port=4
  Circumduction_GuidanceForce : Inport  Port=5
  CalculateStiffnessForOneJoint : LopesDevelopmentLibrary/BlocksForInternalUse/GaitGeneration/CalculateStiffnessForOneJoint
  Constant : Constant  Value=LopesParams.GaitData.StiffnessParameters.HA_WeightShift
  Constant1 : Constant  Value=LopesParams.GaitData.StiffnessParameters.HA_Circumduction
  Mux : Mux  Inputs=2
  Mux1 : Mux  Inputs=2
  TrajectoryOfInfluence : LopesDevelopmentLibrary/BlocksForInternalUse/GaitGeneration/TrajectoryOfInfluence
  TrajectoryOfInfluence1 : LopesDevelopmentLibrary/BlocksForInternalUse/GaitGeneration/TrajectoryOfInfluence
  Stiffness_pct : Outport
  wires:
  CalculateStiffnessForOneJoint/1 -> Stiffness_pct/1
  General_GuidanceForce/1 -> CalculateStiffnessForOneJoint/1
  Constant1/1 -> TrajectoryOfInfluence1/1
  WeightShift_GuidanceForce/1 -> Mux1/1
  Constant/1 -> TrajectoryOfInfluence/1
  breaks/1 -> TrajectoryOfInfluence/2, TrajectoryOfInfluence1/2
  phase/1 -> TrajectoryOfInfluence/3, TrajectoryOfInfluence1/3
  TrajectoryOfInfluence/1 -> Mux/1
  TrajectoryOfInfluence1/1 -> Mux/2
  Circumduction_GuidanceForce/1 -> Mux1/2
  Mux/1 -> CalculateStiffnessForOneJoint/2
  Mux1/1 -> CalculateStiffnessForOneJoint/3

== system LopesDevelopmentLibrary/GaitGeneration/CalculateReferenceStiffnesses/LHF ==
  General_GuidanceForce : Inport
  breaks : Inport  Port=2
  phase : Inport  Port=3
  FootPlacement_GuidanceForce : Inport  Port=4
  StepLength_GuidanceForce : Inport  Port=5
  CalculateStiffnessForOneJoint : LopesDevelopmentLibrary/BlocksForInternalUse/GaitGeneration/CalculateStiffnessForOneJoint
  Constant : Constant  Value=LopesParams.GaitData.StiffnessParameters.HF_FootPlacement
  Constant1 : Constant  Value=LopesParams.GaitData.StiffnessParameters.HF_StepLength
  Mux : Mux  Inputs=2
  Mux1 : Mux  Inputs=2
  TrajectoryOfInfluence : LopesDevelopmentLibrary/BlocksForInternalUse/GaitGeneration/TrajectoryOfInfluence
  TrajectoryOfInfluence1 : LopesDevelopmentLibrary/BlocksForInternalUse/GaitGeneration/TrajectoryOfInfluence
  Stiffness_pct : Outport
  wires:
  Mux1/1 -> CalculateStiffnessForOneJoint/3
  Mux/1 -> CalculateStiffnessForOneJoint/2
  StepLength_GuidanceForce/1 -> Mux1/2
  TrajectoryOfInfluence1/1 -> Mux/2
  TrajectoryOfInfluence/1 -> Mux/1
  phase/1 -> TrajectoryOfInfluence1/3, TrajectoryOfInfluence/3
  breaks/1 -> TrajectoryOfInfluence1/2, TrajectoryOfInfluence/2
  Constant/1 -> TrajectoryOfInfluence/1
  FootPlacement_GuidanceForce/1 -> Mux1/1
  Constant1/1 -> TrajectoryOfInfluence1/1
  General_GuidanceForce/1 -> CalculateStiffnessForOneJoint/1
  CalculateStiffnessForOneJoint/1 -> Stiffness_pct/1

== system LopesDevelopmentLibrary/GaitGeneration/CalculateReferenceStiffnesses/LKF ==
  General_GuidanceForce : Inport
  breaks : Inport  Port=2
  phase : Inport  Port=3
  StepHeight_GuidanceForce : Inport  Port=4
  StabilityInStance_GuidanceForce : Inport  Port=5
  FootPlacement_GuidanceForce : Inport  Port=6
  CalculateStiffnessForOneJoint : LopesDevelopmentLibrary/BlocksForInternalUse/GaitGeneration/CalculateStiffnessForOneJoint
  Constant : Constant  Value=LopesParams.GaitData.StiffnessParameters.KF_StepHeight
  Constant1 : Constant  Value=LopesParams.GaitData.StiffnessParameters.KF_StabilityStance
  Constant2 : Constant  Value=LopesParams.GaitData.StiffnessParameters.KF_FootPlacement
  Mux : Mux  Inputs=3
  Mux1 : Mux  Inputs=3
  TrajectoryOfInfluence : LopesDevelopmentLibrary/BlocksForInternalUse/GaitGeneration/TrajectoryOfInfluence
  TrajectoryOfInfluence1 : LopesDevelopmentLibrary/BlocksForInternalUse/GaitGeneration/TrajectoryOfInfluence
  TrajectoryOfInfluence2 : LopesDevelopmentLibrary/BlocksForInternalUse/GaitGeneration/TrajectoryOfInfluence
  Stiffness_pct : Outport
  wires:
  Mux1/1 -> CalculateStiffnessForOneJoint/3
  Mux/1 -> CalculateStiffnessForOneJoint/2
  StabilityInStance_GuidanceForce/1 -> Mux1/2
  Constant1/1 -> TrajectoryOfInfluence1/1
  TrajectoryOfInfluence1/1 -> Mux/2
  TrajectoryOfInfluence/1 -> Mux/1
  General_GuidanceForce/1 -> CalculateStiffnessForOneJoint/1
  CalculateStiffnessForOneJoint/1 -> Stiffness_pct/1
  StepHeight_GuidanceForce/1 -> Mux1/1
  Constant/1 -> TrajectoryOfInfluence/1
  breaks/1 -> TrajectoryOfInfluence2/2, TrajectoryOfInfluence1/2, TrajectoryOfInfluence/2
  phase/1 -> TrajectoryOfInfluence2/3, TrajectoryOfInfluence1/3, TrajectoryOfInfluence/3
  FootPlacement_GuidanceForce/1 -> Mux1/3
  Constant2/1 -> TrajectoryOfInfluence2/1
  TrajectoryOfInfluence2/1 -> Mux/3

== system LopesDevelopmentLibrary/GaitGeneration/CalculateReferenceStiffnesses/PX ==
  General_GuidanceForce : Inport
  Stiffness_pct : Outport
  wires:
  General_GuidanceForce/1 -> Stiffness_pct/1

== system LopesDevelopmentLibrary/GaitGeneration/CalculateReferenceStiffnesses/PZ ==
  note: We don't need the general guidance force here. If no special
      | attention is paid to the weightshift, it will have the same value as the
      | general guidance force anyway.
  General_GuidanceForce : Inport
  WeightShift_GuidanceForce : Inport  Port=2
  Terminator : Terminator
  Stiffness_pct : Outport
  wires:
  General_GuidanceForce/1 -> Terminator/1
  WeightShift_GuidanceForce/1 -> Stiffness_pct/1

== system LopesDevelopmentLibrary/GaitGeneration/CalculateReferenceStiffnesses/RAP ==
  General_GuidanceForce : Inport
  breaks : Inport  Port=2
  phase : Inport  Port=3
  StepHeight_GuidanceForce : Inport  Port=4
  FootPlacement_GuidanceForce : Inport  Port=5
  PushOff_GuidanceForce : Inport  Port=6
  CalculateStiffnessForOneJoint : LopesDevelopmentLibrary/BlocksForInternalUse/GaitGeneration/CalculateStiffnessForOneJoint
  Constant : Constant  Value=LopesParams.GaitData.StiffnessParameters.AP_StepHeight
  Constant1 : Constant  Value=LopesParams.GaitData.StiffnessParameters.AP_FootPlacement
  Constant2 : Constant  Value=LopesParams.GaitData.StiffnessParameters.AP_PushOff
  Mux : Mux  Inputs=3
  Mux1 : Mux  Inputs=3
  TrajectoryOfInfluence : LopesDevelopmentLibrary/BlocksForInternalUse/GaitGeneration/TrajectoryOfInfluence
  TrajectoryOfInfluence1 : LopesDevelopmentLibrary/BlocksForInternalUse/GaitGeneration/TrajectoryOfInfluence
  TrajectoryOfInfluence2 : LopesDevelopmentLibrary/BlocksForInternalUse/GaitGeneration/TrajectoryOfInfluence
  Stiffness_pct : Outport
  wires:
  Mux1/1 -> CalculateStiffnessForOneJoint/3
  General_GuidanceForce/1 -> CalculateStiffnessForOneJoint/1
  Mux/1 -> CalculateStiffnessForOneJoint/2
  TrajectoryOfInfluence2/1 -> Mux/3
  TrajectoryOfInfluence1/1 -> Mux/2
  TrajectoryOfInfluence/1 -> Mux/1
  PushOff_GuidanceForce/1 -> Mux1/3
  Constant2/1 -> TrajectoryOfInfluence2/1
  FootPlacement_GuidanceForce/1 -> Mux1/2
  Constant1/1 -> TrajectoryOfInfluence1/1
  CalculateStiffnessForOneJoint/1 -> Stiffness_pct/1
  StepHeight_GuidanceForce/1 -> Mux1/1
  Constant/1 -> TrajectoryOfInfluence/1
  breaks/1 -> TrajectoryOfInfluence/2, TrajectoryOfInfluence1/2, TrajectoryOfInfluence2/2
  phase/1 -> TrajectoryOfInfluence/3, TrajectoryOfInfluence1/3, TrajectoryOfInfluence2/3

== system LopesDevelopmentLibrary/GaitGeneration/CalculateReferenceStiffnesses/RHA ==
  WeightShift_GuidanceForce : Inport
  Stiffness_pct : Outport
  wires:
  WeightShift_GuidanceForce/1 -> Stiffness_pct/1
